simulink model "plant_simulation"  (R2020b)
settings: Solver=ode1  StartTime=0.0  StopTime=final_Time  FixedStep=1e-3  RelTol=1e-3
values from neighbouring files (symbols this model uses):
  A_plant = -5    [setup_and_solver.m]
  B_plant = 1    [setup_and_solver.m]
  initial_State_Value = 1    [setup_and_solver.m]
settings Model: Creator=alkim  LastModifiedBy=alkim

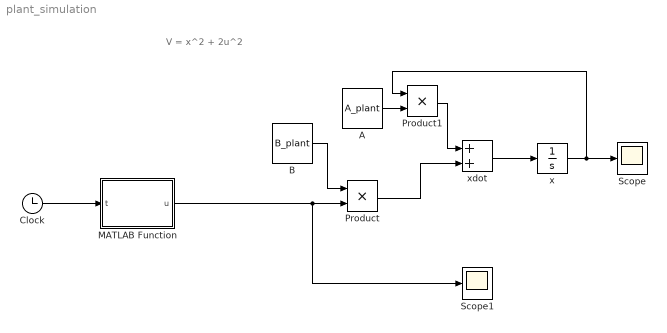
== system plant_simulation ==
  note: V = x^2 + 2u^2
  A : Constant  Value=A_plant
  B : Constant  Value=B_plant
  Clock : Clock
  MATLAB Function : MATLAB Function  TreatAsAtomicUnit=on
  Product : Product
  Product1 : Product
  Scope : Scope
  Scope1 : Scope
  x : Integrator  InitialCondition=initial_State_Value
  xdot : Sum
  wires:
  Product/1 -> xdot/2
  B/1 -> Product/1
  MATLAB Function/1(u) -> Scope1/1, Product/2
  Clock/1 -> MATLAB Function/1(t)
  xdot/1 -> x/1
  x/1 -> Product1/1, Scope/1
  A/1 -> Product1/2
  Product1/1 -> xdot/1

== matlab function plant_simulation/MATLAB Function ==
  data: t input; u output
function u = fcn(t)

u = (exp(sqrt(1.02e+2).*t.*(-1.0./2.0)).*(exp(sqrt(1.02e+2).*t)-exp(sqrt(1.02e+2))).*-5.0)./(exp(sqrt(1.02e+2))-1.0)-(sqrt(1.02e+2).*exp(sqrt(1.02e+2).*t).*exp(sqrt(1.02e+2).*t.*(-1.0./2.0)))./(exp(sqrt(1.02e+2))-1.0)+(sqrt(1.02e+2).*exp(sqrt(1.02e+2).*t.*(-1.0./2.0)).*(exp(sqrt(1.02e+2).*t)-exp(sqrt(1.02e+2))))./(exp(sqrt(1.02e+2)).*2.0-2.0);
